simulink model "cc"  (R2018a)
settings: Solver=VariableStepAuto  StartTime=0.0  StopTime=inf  RelTol=1e-3
values from neighbouring files (symbols this model uses):
  cmd = receive(sub_cmd,1)    [car_env.m]
  lr = 1    [data_vehicle.mat]    (also in golf_car.mat = 1.15)
  m = 1575    [data_vehicle.mat]    (also in golf_car.mat)
  yaw0_ego = egoCar.Yaw    [car_env.m]    (also in data_vehicle.mat = -8.2787154124e-05; golf_car.mat = -8.2787154124e-05; tess2.m)
undefined symbols (not defined in the file or in its folder): Angular, Linear
libraries: robotlib x3, autolibshared x1
settings Model: Creator=allen  LastModifiedBy=allen

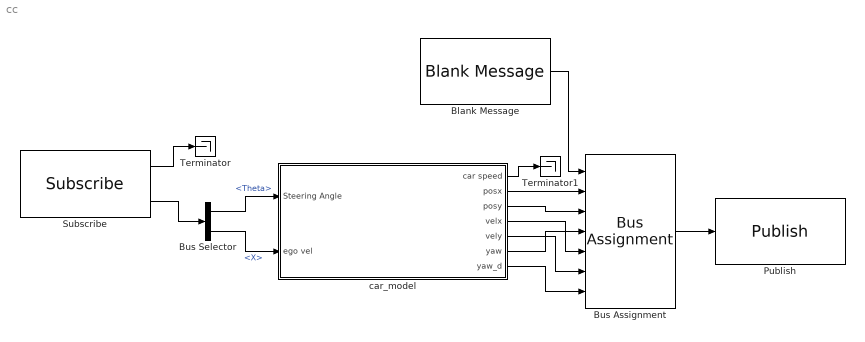
== system cc ==
  Blank Message : robotlib/Blank Message  SourceLibraryInfo=This block requires Robotics System Toolbox  messageType=geometry_msgs/Twist  SampleTime=inf
      settings: SourceProductBaseCode=RO
  Bus Assignment : BusAssignment  AssignedSignals=Linear.X,Linear.Y,Linear.Z,Angular.X,Angular.Y,Angular.Z
  Bus Selector : BusSelector  OutputSignals=Theta,X
  Publish : robotlib/Publish  SourceLibraryInfo=This block requires Robotics System Toolbox  topicSource=Specify your own  topic=/car_info  messageType=geometry_msgs/Twist  messageQueueLength=1
      settings: SourceProductBaseCode=RO
  Subscribe : robotlib/Subscribe  SourceLibraryInfo=This block requires Robotics System Toolbox  topicSource=Specify your own  topic=/cmd  messageType=geometry_msgs/Pose2D  sampleTime=-1  messageQueueLength=1
      settings: SourceProductBaseCode=RO
  Terminator : Terminator
  Terminator1 : Terminator
  car_model : Subsystem
  wires:
  car_model/7(yaw_d) -> Bus Assignment/7
  car_model/2(posx) -> Bus Assignment/2
  car_model/5(vely) -> Bus Assignment/6
  Bus Selector/1 -> car_model/1(Steering Angle)  "<Theta>"
  car_model/4(velx) -> Bus Assignment/5
  Bus Selector/2 -> car_model/2(ego vel)  "<X>"
  car_model/6(yaw) -> Bus Assignment/4
  Blank Message/1 -> Bus Assignment/1
  car_model/3(posy) -> Bus Assignment/3
  car_model/1("car speed ") -> Terminator1/1
  Subscribe/2 -> Bus Selector/1
  Bus Assignment/1 -> Publish/1
  Subscribe/1 -> Terminator/1

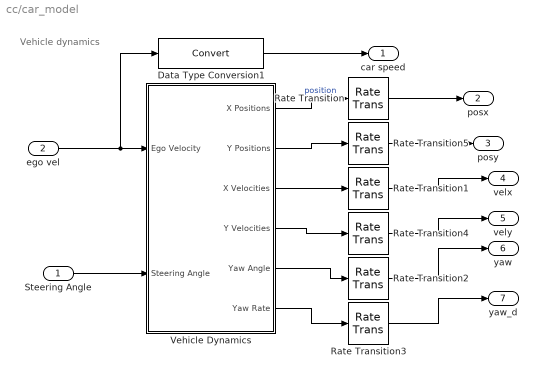
== system cc/car_model ==
  note: Vehicle dynamics
  Steering Angle : Inport  Unit=rad
  ego vel : Inport  Port=2  Unit=m/s
  Data Type Conversion1 : DataTypeConversion
  Rate Transition{,1..5} (6 alike) : RateTransition  OutPortSampleTime=Ts
  Vehicle Dynamics : Subsystem  VariantControl=VariantVDBS
  "car speed " : Outport  OutDataTypeStr=single  Unit=m/s
  posx : Outport  Port=2  Unit=m
  posy : Outport  Port=3  Unit=m
  velx : Outport  Port=4  Unit=m/s
  vely : Outport  Port=5  Unit=m/s
  yaw : Outport  Port=6  Unit=deg
  yaw_d : Outport  Port=7  Unit=deg/s
  wires:
  Vehicle Dynamics/1(X Positions) -> Rate Transition/1  "position"
  Rate Transition1/1 -> velx/1
  ego vel/1 -> Vehicle Dynamics/1(Ego Velocity), Data Type Conversion1/1
  Steering Angle/1 -> Vehicle Dynamics/2(Steering Angle)
  Vehicle Dynamics/6(Yaw Rate) -> Rate Transition3/1
  Vehicle Dynamics/3(X Velocities) -> Rate Transition1/1
  Rate Transition3/1 -> yaw_d/1
  Data Type Conversion1/1 -> "car speed "/1
  Vehicle Dynamics/5(Yaw Angle) -> Rate Transition2/1
  Rate Transition2/1 -> yaw/1
  Vehicle Dynamics/4(Y Velocities) -> Rate Transition4/1
  Vehicle Dynamics/2(Y Positions) -> Rate Transition5/1
  Rate Transition/1 -> posx/1
  Rate Transition5/1 -> posy/1
  Rate Transition4/1 -> vely/1

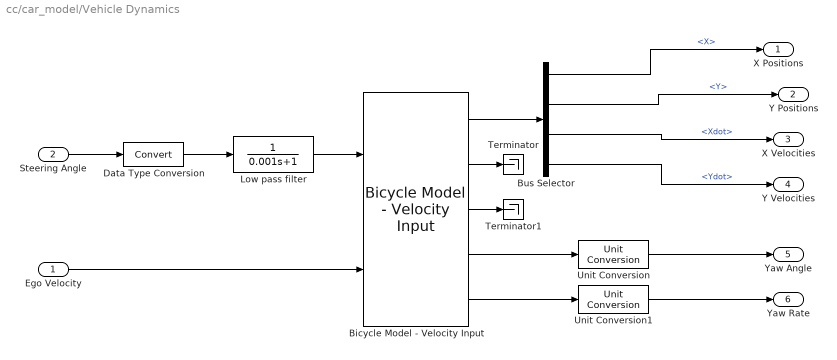
== system cc/car_model/Vehicle Dynamics ==
  Ego Velocity : Inport
  Steering Angle : Inport  Port=2
  Bicycle Model - Velocity Input : autolibshared/Bicycle Model - Velocity Input  trackMode=Single (bicycle)  inputMode=External longitudinal forces  frontSteerMode=on  rearSteerMode=off  windMode=off  muMode=off  extFMode=off  extMMode=off  aMode=3  NF=2  NR=2  m=m  a=lf  b=lr  h=0.35  X_o=x0_ego  xdot_o=0  CalphaMode=off  sigmaMode=on  w=[1.4,1.4]  Cy_f=Cf  Cy_r=Cr  sigma_f=.1  sigma_r=.1  alpha_f_brk=[-.1 .1]  Cy_f_data=[-9e3 9e3]  alpha_r_brk=[-.1 .1]  Cy_r_data=[-9e3 9e3]  Y_o=y0_ego  ydot_o=0  Izz=Iz  psi_o=yaw0_ego*pi/180  r_o=0  Af=2  Cd=.3  Cl=.1  Cpm=.1  beta_w=[0:0.01:0.3]  Cs=[0:0.03:0.9]  Cym=[0:0.01:0.3]  Pabs=101325  Tair=273  g=9.81  mu=1  xdot_tol=.01  Fznom=5000  Fxtire_sat=1e6  Fytire_sat=1e6
      settings: SourceProductName=Powertrain Blockset  SourceProductBaseCode=PW
  Bus Selector : BusSelector  OutputSignals=InertFrm.FrntAxl.Disp.X,InertFrm.FrntAxl.Disp.Y,InertFrm.FrntAxl.Vel.Xdot,InertFrm.FrntAxl.Vel.Ydot
  Data Type Conversion : DataTypeConversion
  Low pass filter : TransferFcn  Denominator=[0.001 1]
  Terminator : Terminator
  Terminator1 : Terminator
  Unit Conversion : UnitConversion  OutputType=Inherit: Inherit via back propagation
  Unit Conversion1 : UnitConversion  OutputType=Inherit: Inherit via back propagation
  X Positions : Outport  Unit=m
  Y Positions : Outport  Port=2  Unit=m
  X Velocities : Outport  Port=3  Unit=m/s
  Y Velocities : Outport  Port=4  Unit=m/s
  Yaw Angle : Outport  Port=5  Unit=deg
  Yaw Rate : Outport  Port=6  Unit=degree/s
  wires:
  Low pass filter/1 -> Bicycle Model - Velocity Input/1
  Steering Angle/1 -> Data Type Conversion/1
  Data Type Conversion/1 -> Low pass filter/1
  Bicycle Model - Velocity Input/3 -> Terminator1/1
  Bicycle Model - Velocity Input/2 -> Terminator/1
  Bus Selector/2 -> Y Positions/1  "<Y>"
  Bus Selector/1 -> X Positions/1  "<X>"
  Bicycle Model - Velocity Input/5 -> Unit Conversion1/1
  Bicycle Model - Velocity Input/4 -> Unit Conversion/1
  Bicycle Model - Velocity Input/1 -> Bus Selector/1
  Ego Velocity/1 -> Bicycle Model - Velocity Input/2
  Unit Conversion/1 -> Yaw Angle/1
  Unit Conversion1/1 -> Yaw Rate/1
  Bus Selector/3 -> X Velocities/1  "<Xdot>"
  Bus Selector/4 -> Y Velocities/1  "<Ydot>"
